simulink model "InnerOuter_Sim_newNav_flightgear_L2"  (Simulink 7.8)
settings: Solver=ode4  StartTime=0.0  StopTime=300  FixedStep=SampleT  RelTol=1e-3
InitFcn:
  | clc
  | innerOuterInit
  | launchFlightgear
values from neighbouring files (symbols this model uses):
  apSampleTime = 0.01    [innerOuterInit.m]
  FLIGHTGEAR_L2_RATE = 10    [launchFlightgear.m]
  SampleT = 0.005    [innerOuterInit.m]
  T = 0.01    [innerOuterInit.m]
undefined symbols (not defined in the file or in its folder): A1, Apolar, bankCommandLimit, baseHeight, BasePoint, baseTemp, CD0, chord, CL0, CLa, CLa_dot, Clb, ClDa, CLDe, CLDf, ClDr, clock, Clp, CLq, Clr, Cm0, Cma, CmDe, CmDf, Cmq, Cnb, CnDa, CnDr, Cnp, Cnr, compensatorOn, CYb, CYDr, da_failamp, da_failbias, da_failper, daL_fail, daR_fail, deg, DiscIntNeverNeededParam, dr_fail, dr_failamp, dr_failbias, dr_failper, Earth, elarm, Euler_0, F, gaind, getGSLocation, getWP, GS_location, Init_onlyOnce, Init_Reset, IPStar, ISA_g, Ixx, Iyy, Izz, L1OF ... (+38)
libraries: simulink x74, SLUGS_Library x41, aerolibconvert2 x24, dsPICdrivers x10, aerolibactuator x5, aerolibtransform2 x4, aerolibobsolete x3, dspmtrx3 x3, aerolibwind2 x2, aerolibfltsims x2, aerolibatmos2 x1, aerolibanimutils x1
(part 2 of 5)

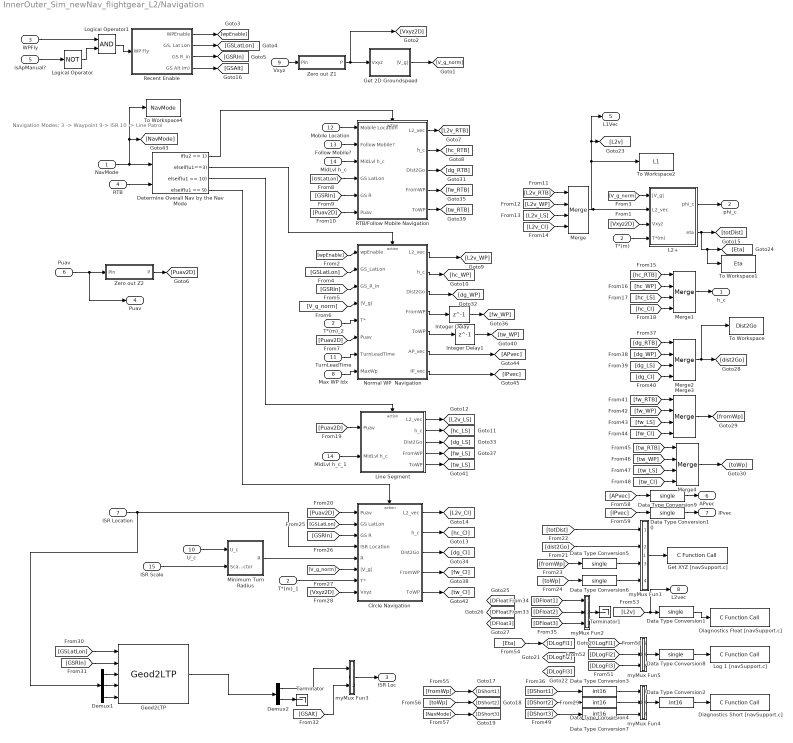
== system InnerOuter_Sim_newNav_flightgear_L2/Navigation ==
  note: Navigation Modes:
      | 3 -> Waypoint
      | 9-> ISR
      | 10 -> Line Patrol
  NavMode : Inport
  T*(m) : Inport  Port=2
  WPFly : Inport  Port=3
  RTB : Inport  Port=4
  isApManual? : Inport  Port=5
  Puav : Inport  Port=6  SampleTime=apSampleTime
  ISR Location : Inport  Port=7
  Max WP Idx : Inport  Port=8
  Vxyz : Inport  Port=9  SampleTime=apSampleTime
  U_c : Inport  Port=10
  TurnLeadTime : Inport  Port=11
  Mobile Location : Inport  Port=12
  Follow Mobile? : Inport  Port=13
  MidLvl h_c : Inport  Port=14
  ISR Scale : Inport  Port=15
  Circle Navigation : Subsystem  TreatAsAtomicUnit=on
  Data Type Conversion{1,5..6,8..10} (6 alike) : DataTypeConversion  OutDataTypeStr=single
  Data Type Conversion{2..4,7} (4 alike) : DataTypeConversion  OutDataTypeStr=int16
  Demux1 : Demux  Outputs=3
  Demux2 : Demux  Outputs=[2 1]
  Determine Overall Nav by the Nav Mode : If  NumInputs=2  IfExpression=u2 == 1  ElseIfExpressions=u1==3, u1 == 10, u1 == 9  ShowElse=off
  Diagnostics Float [navSupport.c] : dsPICdrivers/OTHERS/C Function Call  Tag=dsPIC_dsPIC_CFunctionCall  FctUpdate=Output Function  fctName='setDiagnosticFloat'  INPUT_SIZE=3  INPUT1=real32  INPUT2=--  INPUT3=--  OUTPUT_SIZE=1  OUTPUT1=--  SampleTime=.01  InputType=[ 7 ]  OutputType=[ ]  FctDeclaration=extern void setDiagnosticFloat(real32_T* u1);  FctCall=setDiagnosticFloat(*%u1);  OrderingInOutPopup=None  FctStart=None  FctStart_Name=Init_onlyOnce  FctStart_Declaration=inline extern void Init_onlyOnce();  FctStart_Call=Init_onlyOnce();  FctInit=None  FctInit_Name=Init_Reset  FctInit_Declaration=inline extern void Init_Reset();  FctInit_Call=Init_Reset();  PinDigitalInput=[]  PinDigitalOutput=[]  AnalogueInput=[]
  Diagnostics Short [navSupport.c] : dsPICdrivers/OTHERS/C Function Call  Tag=dsPIC_dsPIC_CFunctionCall  FctUpdate=Output Function  fctName='setDiagnosticShort'  INPUT_SIZE=3  INPUT1=int16  INPUT2=--  INPUT3=--  OUTPUT_SIZE=1  OUTPUT1=--  SampleTime=.01  InputType=[ 3 ]  OutputType=[ ]  FctDeclaration=extern void setDiagnosticShort(int16_T* u1);  FctCall=setDiagnosticShort(*%u1);  OrderingInOutPopup=None  FctStart=None  FctStart_Name=Init_onlyOnce  FctStart_Declaration=inline extern void Init_onlyOnce();  FctStart_Call=Init_onlyOnce();  FctInit=None  FctInit_Name=Init_Reset  FctInit_Declaration=inline extern void Init_Reset();  FctInit_Call=Init_Reset();  PinDigitalInput=[]  PinDigitalOutput=[]  AnalogueInput=[]
  Geod2LTP : SLUGS_Library/Navigation/Geod2LTP
  Get 2D Groundspeed : Subsystem
  Get XYZ [navSupport.c] : dsPICdrivers/OTHERS/C Function Call  Tag=dsPIC_dsPIC_CFunctionCall  FctUpdate=Output Function  fctName='setNavNav'  INPUT_SIZE=4  INPUT1=real32  INPUT2=--  INPUT3=--  OUTPUT_SIZE=1  OUTPUT1=--  SampleTime=.01  InputType=[ 7 ]  OutputType=[ ]  FctDeclaration=extern void setNavNav(real32_T* u1);  FctCall=setNavNav(*%u1);  OrderingInOutPopup=None  FctStart=None  FctStart_Name=Init_onlyOnce  FctStart_Declaration=inline extern void Init_onlyOnce();  FctStart_Call=Init_onlyOnce();  FctInit=None  FctInit_Name=Init_Reset  FctInit_Declaration=inline extern void Init_Reset();  FctInit_Call=Init_Reset();  PinDigitalInput=[]  PinDigitalOutput=[]  AnalogueInput=[]
  Integer Delay : Delay  DelayLength=1  InputProcessing=Inherited
  Integer Delay1 : Delay  DelayLength=1  InputProcessing=Inherited
  L2+ : Subsystem
  Line Segment : Subsystem  TreatAsAtomicUnit=on
  Log 1 [navSupport.c] : dsPICdrivers/OTHERS/C Function Call  Tag=dsPIC_dsPIC_CFunctionCall  FctUpdate=Output Function  fctName='setLogFloat1'  INPUT_SIZE=3  INPUT1=real32  INPUT2=--  INPUT3=--  OUTPUT_SIZE=1  OUTPUT1=--  SampleTime=.01  InputType=[ 7 ]  OutputType=[ ]  FctDeclaration=extern void setLogFloat1(real32_T* u1);  FctCall=setLogFloat1(*%u1);  OrderingInOutPopup=None  FctStart=None  FctStart_Name=Init_onlyOnce  FctStart_Declaration=inline extern void Init_onlyOnce();  FctStart_Call=Init_onlyOnce();  FctInit=None  FctInit_Name=Init_Reset  FctInit_Declaration=inline extern void Init_Reset();  FctInit_Call=Init_Reset();  PinDigitalInput=[]  PinDigitalOutput=[]  AnalogueInput=[]
  Logical Operator : Logic  Operator=NOT  AllPortsSameDT=off  OutDataTypeStr=boolean
  Logical Operator1 : Logic  AllPortsSameDT=off  OutDataTypeStr=boolean
  Merge{,1..4} (5 alike) : Merge  Inputs=4
  MidLvl h_c_1 : InportShadow  Port=14
  Minimum Turn Radius : Subsystem
  Normal WP  Navigation : Subsystem  TreatAsAtomicUnit=on
  RTB/Follow Mobile Navigation : Subsystem
  Recent Enable : Subsystem
  T*(m)_1 : InportShadow  Port=2
  T*(m)_2 : InportShadow  Port=2
  Terminator : Terminator
  Terminator1 : Terminator
  To Workspace : ToWorkspace  VariableName=Dist2Go  SampleTime=-1  SaveFormat=Array
  To Workspace1 : ToWorkspace  VariableName=Eta  SampleTime=-1  SaveFormat=Array
  To Workspace2 : ToWorkspace  VariableName=L1  SampleTime=-1  SaveFormat=Array
  To Workspace4 : ToWorkspace  VariableName=NavMode  SampleTime=-1  SaveFormat=Array
  Zero out Z1 : MATLAB Function  TreatAsAtomicUnit=on
  Zero out Z2 : MATLAB Function  TreatAsAtomicUnit=on
  myMux Fun1 : MATLAB Function  TreatAsAtomicUnit=on
  myMux Fun2 : MATLAB Function  TreatAsAtomicUnit=on
  myMux Fun3 : MATLAB Function  TreatAsAtomicUnit=on
  myMux Fun4 : MATLAB Function  TreatAsAtomicUnit=on
  myMux Fun5 : MATLAB Function  TreatAsAtomicUnit=on
  h_c : Outport
  phi_c : Outport  Port=2
  ISR Loc : Outport  Port=3
  "Puav " : Outport  Port=4
  L1Vec : Outport  Port=5
  APvec : Outport  Port=6
  IPvec : Outport  Port=7
  L2vec : Outport  Port=8
  wires:
  ? -> [DLogFl3]
  ? -> [DLogFl2]
  myMux Fun2/1(y) -> Terminator1/1
  ? -> [DFloat1]
  [NavMode] -> [DShort3]
  [toWp] -> [DShort2]
  [fromWp] -> [DShort1]
  [Eta] -> [DLogFl1]
  [L2v] -> Data Type Conversion1/1, L2vec/1
  Data Type Conversion8/1 -> Log 1 [navSupport.c]/1
  [DLogFl1] -> myMux Fun5/1(u1)
  [DLogFl2] -> myMux Fun5/2(u2)
  [DLogFl3] -> myMux Fun5/3(u3)
  myMux Fun5/1(y) -> Data Type Conversion8/1
  Data Type Conversion7/1 -> myMux Fun4/3(u3)
  Data Type Conversion4/1 -> myMux Fun4/2(u2)
  Data Type Conversion3/1 -> myMux Fun4/1(u1)
  [DShort3] -> Data Type Conversion7/1
  [DShort1] -> Data Type Conversion3/1
  [DShort2] -> Data Type Conversion4/1
  myMux Fun4/1(y) -> Data Type Conversion2/1
  Data Type Conversion2/1 -> Diagnostics Short [navSupport.c]/1
  [GSAlt] -> myMux Fun3/2(u2)
  Geod2LTP/1 -> Demux2/1
  Demux2/2 -> Terminator/1
  Demux2/1 -> myMux Fun3/1(u1)
  myMux Fun3/1(y) -> ISR Loc/1
  [GSRIn] -> Geod2LTP/2
  [GSLatLon] -> Geod2LTP/1
  Demux1/3 -> Geod2LTP/5
  Demux1/2 -> Geod2LTP/4
  Demux1/1 -> Geod2LTP/3
  Data Type Conversion1/1 -> Diagnostics Float [navSupport.c]/1
  [DFloat3] -> myMux Fun2/3(u3)
  [DFloat1] -> myMux Fun2/1(u1)
  [DFloat2] -> myMux Fun2/2(u2)
  ISR Scale/1 -> Minimum Turn Radius/2(Scale Factor)
  Recent Enable/4(GS Alt (m)) -> [GSAlt]
  Determine Overall Nav by the Nav Mode/3 -> Line Segment/Action
  U_c/1 -> Minimum Turn Radius/1(U_c)
  ISR Location/1 -> Demux1/1, Circle Navigation/4(ISR Location)
  [Vxyz2D] -> Circle Navigation/8(Vxyz)
  T*(m)_1/1 -> Circle Navigation/7(T*)
  [V_g_norm] -> Circle Navigation/6(|V_g|)
  Minimum Turn Radius/1(R) -> Circle Navigation/5(R)
  [GSRIn] -> Circle Navigation/3(GS R)
  [GSLatLon] -> Circle Navigation/2(GS LatLon)
  Circle Navigation/5(ToWP) -> [tw_CI]
  Circle Navigation/4(FromWP) -> [fw_CI]
  Circle Navigation/3(Dist2Go) -> [dg_CI]
  Circle Navigation/1(L2_vec) -> [L2v_CI]
  Circle Navigation/2(h_c) -> [hc_CI]
  [Puav2D] -> Circle Navigation/1(Puav)
  Integer Delay1/1 -> [tw_WP]
  Integer Delay/1 -> [fw_WP]
  Line Segment/5(ToWP) -> [tw_LS]
  RTB/Follow Mobile Navigation/5(ToWP) -> [tw_RTB]
  Line Segment/4(FromWP) -> [fw_LS]
  Normal WP  Navigation/4(FromWP) -> Integer Delay/1
  RTB/Follow Mobile Navigation/4(FromWP) -> [fw_RTB]
  Line Segment/3(Dist2Go) -> [dg_LS]
  Normal WP  Navigation/3(Dist2Go) -> [dg_WP]
  RTB/Follow Mobile Navigation/3(Dist2Go) -> [dg_RTB]
  Merge3/1 -> [fromWp]
  Merge4/1 -> [toWp]
  Merge2/1 -> [dist2Go], To Workspace/1
  [tw_RTB] -> Merge4/1
  [tw_WP] -> Merge4/2
  [tw_LS] -> Merge4/3
  [tw_CI] -> Merge4/4
  [fw_RTB] -> Merge3/1
  [fw_WP] -> Merge3/2
  [fw_LS] -> Merge3/3
  [fw_CI] -> Merge3/4
  [dg_RTB] -> Merge2/1
  [dg_WP] -> Merge2/2
  [dg_LS] -> Merge2/3
  [dg_CI] -> Merge2/4
  L2+/2(eta) -> [totDist], [Eta], To Workspace1/1
  Data Type Conversion6/1 -> myMux Fun1/4(u4)
  Data Type Conversion5/1 -> myMux Fun1/3(u3)
  [toWp] -> Data Type Conversion6/1
  [fromWp] -> Data Type Conversion5/1
  [dist2Go] -> myMux Fun1/2(u2)
  [totDist] -> myMux Fun1/1(u1)
  myMux Fun1/1(y) -> Get XYZ [navSupport.c]/1
  Vxyz/1 -> Zero out Z1/1(Pin)
  Get 2D Groundspeed/1(|V_g|) -> [V_g_norm]
  [Vxyz2D] -> L2+/3(Vxyz)
  [V_g_norm] -> L2+/1(|V_g|)
  L2+/1(phi_c) -> phi_c/1
  T*(m)/1 -> L2+/4(T*(m))
  NavMode/1 -> Determine Overall Nav by the Nav Mode/1, [NavMode], To Workspace4/1
  Merge/1 -> L2+/2(L2_vec), To Workspace2/1, [L2v], L1Vec/1
  Recent Enable/1(WPEnable) -> [wpEnable]
  Recent Enable/2("GS, Lat Lon") -> [GSLatLon]
  Recent Enable/3(GS R_in) -> [GSRIn]
  Determine Overall Nav by the Nav Mode/2 -> Normal WP  Navigation/Action
  Determine Overall Nav by the Nav Mode/4 -> Circle Navigation/Action
  RTB/1 -> Determine Overall Nav by the Nav Mode/2
  Follow Mobile?/1 -> RTB/Follow Mobile Navigation/2(Follow Mobile?)
  MidLvl h_c/1 -> RTB/Follow Mobile Navigation/3(MidLvl h_c)
  Mobile Location/1 -> RTB/Follow Mobile Navigation/1(Mobile Location)
  Determine Overall Nav by the Nav Mode/1 -> RTB/Follow Mobile Navigation/Action
  Zero out Z1/1(P) -> Get 2D Groundspeed/1(Vxyz), [Vxyz2D]
  Puav/1 -> "Puav "/1, Zero out Z2/1(Pin)
  [GSRIn] -> Normal WP  Navigation/3(GS_R_in)
  [GSLatLon] -> Normal WP  Navigation/2(GS_LatLon)
  [wpEnable] -> Normal WP  Navigation/1(wpEnable)
  [V_g_norm] -> Normal WP  Navigation/4(|V_g|)
  T*(m)_2/1 -> Normal WP  Navigation/5(T*)
  [Puav2D] -> Normal WP  Navigation/6(Puav)
  TurnLeadTime/1 -> Normal WP  Navigation/7(TurnLeadTime)
  Max WP Idx/1 -> Normal WP  Navigation/8(MaxWp)
  [GSLatLon] -> RTB/Follow Mobile Navigation/4(GS LatLon)
  [GSRIn] -> RTB/Follow Mobile Navigation/5(GS R)
  Zero out Z2/1(P) -> [Puav2D]
  [Puav2D] -> RTB/Follow Mobile Navigation/6(Puav)
  Merge1/1 -> h_c/1
  RTB/Follow Mobile Navigation/1(L2_vec) -> [L2v_RTB]
  RTB/Follow Mobile Navigation/2(h_c) -> [hc_RTB]
  Normal WP  Navigation/1(L2_vec) -> [L2v_WP]
  Normal WP  Navigation/2(h_c) -> [hc_WP]
  Line Segment/1(L2_vec) -> [L2v_LS]
  Line Segment/2(h_c) -> [hc_LS]
  [L2v_RTB] -> Merge/1
  [L2v_WP] -> Merge/2
  [L2v_LS] -> Merge/3
  [L2v_CI] -> Merge/4
  [hc_RTB] -> Merge1/1
  [hc_WP] -> Merge1/2
  [hc_LS] -> Merge1/3
  [hc_CI] -> Merge1/4
  [Puav2D] -> Line Segment/1(Puav)
  MidLvl h_c_1/1 -> Line Segment/2(MidLvl h_c)
  isApManual?/1 -> Logical Operator/1
  Logical Operator1/1 -> Recent Enable/1(WP Fly)
  Logical Operator/1 -> Logical Operator1/2
  WPFly/1 -> Logical Operator1/1
  Normal WP  Navigation/5(ToWP) -> Integer Delay1/1
  Normal WP  Navigation/6(AP_vec) -> [APvec]
  [APvec] -> Data Type Conversion9/1
  Data Type Conversion9/1 -> APvec/1
  Normal WP  Navigation/7(IP_vec) -> [IPvec]
  [IPvec] -> Data Type Conversion10/1
  Data Type Conversion10/1 -> IPvec/1

== system InnerOuter_Sim_newNav_flightgear_L2/PT Unit (Mariano) ==
  Rb2g : Inport
  cor_b : Inport  Port=2
  Puav : Inport  Port=3
  ISR Location : Inport  Port=4
  Divide : Product  Inputs=*/
  Normalize : Product  Inputs=*/
  Product1 : Product  Multiplication=Matrix(*)  RndMeth=Zero
  Product2 : Product  Multiplication=Matrix(*)  RndMeth=Zero
  Subtract2 : Sum  Inputs=--+
  Transpose1 : dspmtrx3/Transpose  Hermitian=off  overflowFlag=off
  Vector Norm : SLUGS_Library/Vector Norm
  "[-90 90]" : Saturate  UpperLimit=1.5708  LowerLimit=-1.5708
  "[-90 90]1" : Saturate  UpperLimit=1.5708  LowerLimit=-1.5708
  "[a b c]" : Demux  Outputs=3
  dsPIC_asin : SLUGS_Library/dsPIC_asin
  dsPIC_atan : SLUGS_Library/dsPIC_atan
  Tilt_c : Outport
  Pan_c : Outport  Port=2
  wires:
  Rb2g/1 -> Transpose1/1, Product2/1  "Tbg"
  cor_b/1 -> Product1/2
  Vector Norm/1 -> Normalize/2
  Normalize/1 -> Product2/2
  Product2/1 -> "[a b c]"/1
  "[a b c]"/3 -> dsPIC_asin/1
  "[a b c]"/2 -> Divide/1
  "[a b c]"/1 -> Divide/2
  Divide/1 -> dsPIC_atan/1
  dsPIC_atan/1 -> "[-90 90]"/1
  Subtract2/1 -> Normalize/1, Vector Norm/1
  Transpose1/1 -> Product1/1
  "[-90 90]"/1 -> Pan_c/1
  "[-90 90]1"/1 -> Tilt_c/1
  dsPIC_asin/1 -> "[-90 90]1"/1
  ISR Location/1 -> Subtract2/3  "Xt"
  Puav/1 -> Subtract2/2  "Xac"
  Product1/1 -> Subtract2/1  "Tgb * cor_b"

== system InnerOuter_Sim_newNav_flightgear_L2/PT Unit (Vlad)  ==
  Euler (Rad) : Inport
  Tgt (NEU) : Inport  Port=2
  Puav (NEU) : Inport  Port=3
  Display1 : Display
  Divide : Product  Inputs=*/
  LPF the Euler and Construct Matrix : Subsystem
  Product1 : Product  Multiplication=Matrix(*)  RndMeth=Zero
  Subtract : Sum  Inputs=+-
  Trigonometric Function1 : Trigonometry  Operator=atan2
  Trigonometric Function2 : Trigonometry  Operator=asin
  Vector Norm : SLUGS_Library/Vector Norm
  "[-1 1]" : Saturate  UpperLimit=1  LowerLimit=-1
  "[-88 0]" : Saturate  UpperLimit=0  LowerLimit=-1.5708
  "[-98 98]" : Saturate  UpperLimit=1.7104  LowerLimit=-1.7104
  "[a b c]" : Demux  Outputs=3
  Tilt (rad) : Outport
  Pan (rad) : Outport  Port=2
  wires:
  Subtract/1 -> Product1/2  "Tgt_WR_UAV  (NEU)"
  LPF the Euler and Construct Matrix/1(Rfg2b) -> Product1/1
  "[a b c]"/2 -> Trigonometric Function1/1
  "[a b c]"/1 -> Trigonometric Function1/2
  Trigonometric Function1/1 -> "[-98 98]"/1
  Trigonometric Function2/1 -> "[-88 0]"/1, Display1/1
  Product1/1 -> "[a b c]"/1, Vector Norm/1
  "[-1 1]"/1 -> Trigonometric Function2/1
  "[a b c]"/3 -> Divide/1
  Vector Norm/1 -> Divide/2
  Divide/1 -> "[-1 1]"/1
  Euler (Rad)/1 -> LPF the Euler and Construct Matrix/1(Euler)
  "[-98 98]"/1 -> Pan (rad)/1
  Tgt (NEU)/1 -> Subtract/1
  "[-88 0]"/1 -> Tilt (rad)/1
  Puav (NEU)/1 -> Subtract/2

== system InnerOuter_Sim_newNav_flightgear_L2/Send IP to Flightgear ==
  IPvec : Inport
  Enable : EnablePort
  Demux8 : Demux  Outputs=2
  First WP Height : Constant  Value=Zpoints(1)  SampleTime=-1
  Flat Earth to LLA1 : aerolibtransform2/Flat Earth to LLA  units=Metric (MKS)  ptype=Earth (WGS84)  F=1/298.257223563  R=6378137  LL0=GS_location(2:3)  psi=0
  MATLAB Function : MATLAB Function  TreatAsAtomicUnit=on
  NEU2NED : Gain  Gain=[ 1 1 -1]'  SaturateOnIntegerOverflow=on  OutDataTypeStr=Inherit: Same as input  ParamDataTypeStr=Inherit: Same as input
  Terminator : Terminator
  Zero level trust : Constant  Value=0  SampleTime=-1
  wires:
  NEU2NED/1 -> Flat Earth to LLA1/1
  Zero level trust/1 -> Flat Earth to LLA1/2
  Demux8/1 -> MATLAB Function/1(ip_lat)
  Demux8/2 -> MATLAB Function/2(ip_lon)
  Flat Earth to LLA1/1 -> Demux8/1
  Flat Earth to LLA1/2 -> Terminator/1
  First WP Height/1 -> MATLAB Function/3(ip_h)
  IPvec/1 -> NEU2NED/1

== system InnerOuter_Sim_newNav_flightgear_L2/Send L2 to Flightgear ==
  L2vec : Inport
  Enable : EnablePort
  Demux : Demux  Outputs=3
  Demux8 : Demux  Outputs=2
  Flat Earth to LLA1 : aerolibtransform2/Flat Earth to LLA  units=Metric (MKS)  ptype=Earth (WGS84)  F=1/298.257223563  R=6378137  LL0=GS_location(2:3)  psi=0
  MATLAB Function : MATLAB Function  TreatAsAtomicUnit=on
  Mux : Mux  Inputs=3
  NEU2NED : Gain  Gain=[ 1 1 -1]'  SaturateOnIntegerOverflow=on  OutDataTypeStr=Inherit: Same as input  ParamDataTypeStr=Inherit: Same as input
  Terminator : Terminator
  Zero level trust : Constant  Value=0  SampleTime=-1
  wires:
  NEU2NED/1 -> Flat Earth to LLA1/1
  Zero level trust/1 -> Flat Earth to LLA1/2
  Flat Earth to LLA1/1 -> Demux8/1
  Flat Earth to LLA1/2 -> Terminator/1
  Demux8/2 -> MATLAB Function/2(l2_lon)
  Demux8/1 -> MATLAB Function/1(l2_lat)
  Demux/3 -> Mux/3
  L2vec/1 -> Demux/1
  Mux/1 -> NEU2NED/1
  Demux/1 -> Mux/1
  Demux/2 -> Mux/2

== system InnerOuter_Sim_newNav_flightgear_L2/Simple Car Model ==
  Heading : Inport
  Speed : Inport  Port=2
  Heading/Speed to Velocity : Subsystem
  Simple Car Model : Subsystem
  basePoint : Outport
  wires:
  Heading/Speed to Velocity/1(Velocity) -> Simple Car Model/1(Velocity)
  Heading/1 -> Heading/Speed to Velocity/1(Heading)
  Simple Car Model/1(p_cg) -> basePoint/1
  Speed/1 -> Heading/Speed to Velocity/2(Speed)

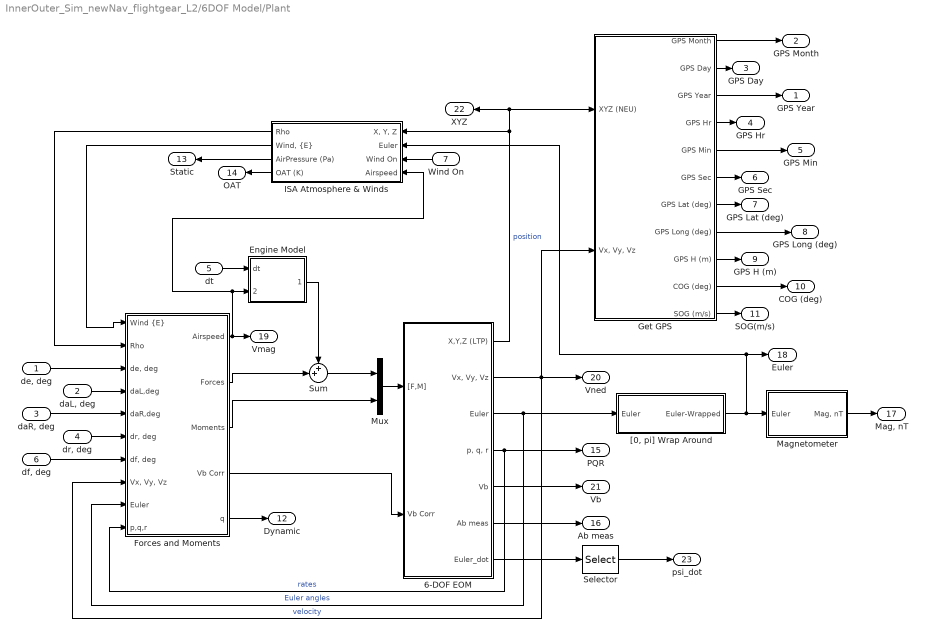
== system InnerOuter_Sim_newNav_flightgear_L2/6DOF Model/Plant ==
  "de, deg" : Inport
  "daL, deg" : Inport  Port=2
  "daR, deg" : Inport  Port=3
  "dr, deg" : Inport  Port=4
  dt : Inport  Port=5
  "df, deg" : Inport  Port=6
  Wind On : Inport  Port=7
  6-DOF EOM : Subsystem
  Engine Model : Subsystem
  Forces and Moments : Subsystem
  Get GPS : Subsystem
  ISA Atmosphere & Winds : Subsystem
  Magnetometer : Subsystem  mask{magField=[ 23143.6 5858.2 45511.9]}
      mask prompts: magField "Local Magnetic Field"
      mask help:
      | Simulates the Data from magnetometers with no noise.
      |
      | You can obtain data for the local magnetic field at:
      |
      | http://www.ngdc.noaa.gov/geomagmodels/IGRFWMM.jsp
  Mux : Mux  Inputs=2
  Selector : Selector  InputPortWidth=3  IndexOptions=Index vector (dialog)  Indices=[3]  OutputSizes=1
  Sum : Sum  Inputs=++|  SaturateOnIntegerOverflow=on
  "[0, pi] Wrap Around" : Subsystem
  GPS Year : Outport
  GPS Month : Outport  Port=2
  GPS Day : Outport  Port=3
  GPS Hr : Outport  Port=4
  GPS Min : Outport  Port=5
  GPS Sec : Outport  Port=6
  GPS Lat (deg) : Outport  Port=7
  GPS Long (deg) : Outport  Port=8
  GPS H (m) : Outport  Port=9
  COG (deg) : Outport  Port=10
  SOG(m/s) : Outport  Port=11
  Dynamic : Outport  Port=12
  Static : Outport  Port=13
  OAT : Outport  Port=14
  PQR : Outport  Port=15
  Ab meas : Outport  Port=16
  "Mag, nT" : Outport  Port=17
  Euler : Outport  Port=18
  Vmag : Outport  Port=19
  Vned : Outport  Port=20
  Vb : Outport  Port=21
  XYZ : Outport  Port=22
  psi_dot : Outport  Port=23
  wires:
  Get GPS/1(GPS Month) -> GPS Month/1
  Get GPS/2(GPS Day) -> GPS Day/1
  Get GPS/3(GPS Year) -> GPS Year/1
  Get GPS/4(GPS Hr) -> GPS Hr/1
  Get GPS/5(GPS Min) -> GPS Min/1
  Get GPS/6(GPS Sec) -> GPS Sec/1
  Get GPS/7(GPS Lat (deg)) -> GPS Lat (deg)/1
  Get GPS/8(GPS Long (deg)) -> GPS Long (deg)/1
  Get GPS/9(GPS H (m)) -> GPS H (m)/1
  6-DOF EOM/6(Ab meas) -> Ab meas/1
  Mux/1 -> 6-DOF EOM/1("[F,M]")
  6-DOF EOM/5(Vb) -> Vb/1
  Engine Model/1(Thrust) -> Sum/1
  Forces and Moments/5(q) -> Dynamic/1
  ISA Atmosphere & Winds/3(AirPressure (Pa)) -> Static/1
  Forces and Moments/1(Airspeed) -> Vmag/1, Engine Model/2(Vmag), ISA Atmosphere & Winds/4(Airspeed)
  ISA Atmosphere & Winds/2("Wind, {E}") -> Forces and Moments/1("Wind {E}")
  ISA Atmosphere & Winds/1(Rho) -> Forces and Moments/2(Rho)
  Forces and Moments/3(Moments) -> Mux/2
  Forces and Moments/2(Forces) -> Sum/2
  Sum/1 -> Mux/1
  Forces and Moments/4(Vb Corr) -> 6-DOF EOM/2(Vb Corr)
  6-DOF EOM/1(X,Y,Z (LTP)) -> ISA Atmosphere & Winds/1("X, Y, Z"), Get GPS/1(XYZ (NEU)), XYZ/1  "position"
  6-DOF EOM/2("Vx, Vy, Vz") -> Vned/1, Get GPS/2("Vx, Vy, Vz"), Forces and Moments/8("Vx, Vy, Vz ")  "velocity"
  6-DOF EOM/3(Euler) -> "[0, pi] Wrap Around"/1(Euler), Forces and Moments/9(Euler)  "Euler angles"
  6-DOF EOM/4("p, q, r") -> PQR/1, Forces and Moments/10(p,q,r)  "rates"
  dt/1 -> Engine Model/1(dt)
  "de, deg"/1 -> Forces and Moments/3("de, deg")
  "daL, deg"/1 -> Forces and Moments/4(daL,deg)
  "dr, deg"/1 -> Forces and Moments/6("dr, deg")
  "df, deg"/1 -> Forces and Moments/7("df, deg")
  "[0, pi] Wrap Around"/1(Euler-Wrapped) -> Magnetometer/1(Euler), Euler/1, ISA Atmosphere & Winds/2(Euler)
  Magnetometer/1("Mag, nT") -> "Mag, nT"/1
  Get GPS/10(COG (deg)) -> COG (deg)/1
  Get GPS/11(SOG (m/s)) -> SOG(m/s)/1
  ISA Atmosphere & Winds/4(OAT (K)) -> OAT/1
  6-DOF EOM/7(Euler_dot) -> Selector/1
  Selector/1 -> psi_dot/1
  Wind On/1 -> ISA Atmosphere & Winds/3(Wind On)
  "daR, deg"/1 -> Forces and Moments/5(daR,deg)

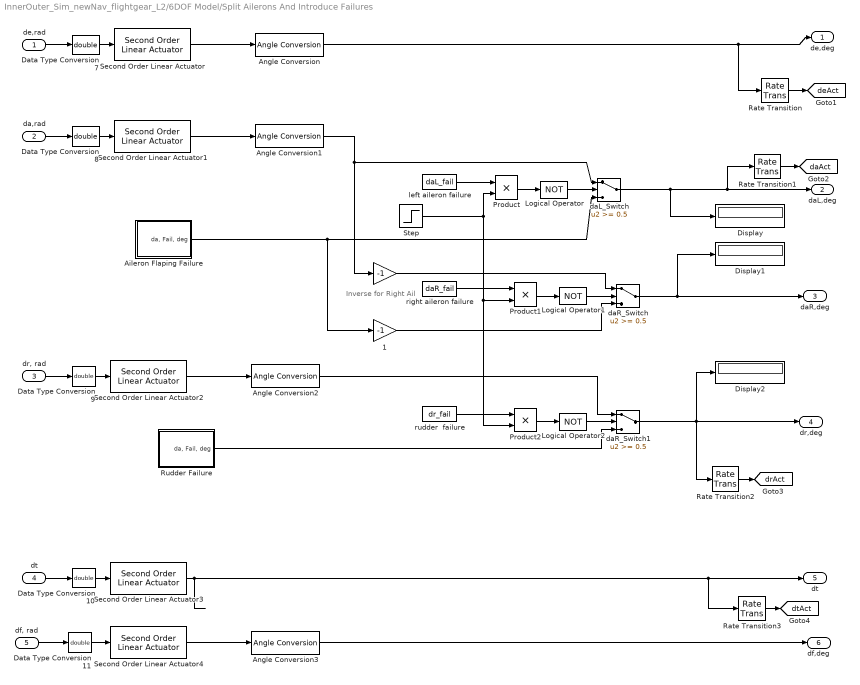
== system InnerOuter_Sim_newNav_flightgear_L2/6DOF Model/Split Ailerons And Introduce Failures ==
  note: Inverse
      | for Right
      | Ail
  de,rad : Inport
  da,rad : Inport  Port=2
  "dr, rad" : Inport  Port=3
  dt : Inport  Port=4
  "df, rad" : Inport  Port=5
  " " : Gain  Gain=-1  SaturateOnIntegerOverflow=on  OutDataTypeStr=Inherit: Same as input  ParamDataTypeStr=Inherit: Same as input
  " 1" : Gain  Gain=-1  SaturateOnIntegerOverflow=on  OutDataTypeStr=Inherit: Same as input  ParamDataTypeStr=Inherit: Same as input
  Aileron Flaping Failure : Subsystem
  Angle Conversion{,1..3} (4 alike) : aerolibconvert2/Angle Conversion  IU=rad  OU=deg
  Data Type Conversion{7..11} (5 alike) : DataTypeConversion  OutDataTypeStr=double
  Display : Display
  Display1 : Display
  Display2 : Display
  Logical Operator : Logic  Operator=NOT  AllPortsSameDT=off  OutDataTypeStr=boolean
  Logical Operator1 : Logic  Operator=NOT  AllPortsSameDT=off  OutDataTypeStr=boolean
  Logical Operator2 : Logic  Operator=NOT  AllPortsSameDT=off  OutDataTypeStr=boolean
  Product : Product  RndMeth=Zero
  Product1 : Product  RndMeth=Zero
  Product2 : Product  RndMeth=Zero
  Rate Transition{,1..3} (4 alike) : RateTransition  OutPortSampleTime=apSampleTime
  Rudder Failure : Subsystem
  Second Order Linear Actuator{,1..3} (4 alike) : aerolibactuator/Second Order Linear Actuator  wn_fin=15  z_fin=0.8  fin_act_0=0
  Second Order Linear Actuator4 : aerolibactuator/Second Order Linear Actuator  wn_fin=150  z_fin=0.7  fin_act_0=0
  Step : Step  Time=tfailure
  daL_Switch : Switch  Threshold=0.5
  daR_Switch : Switch  Threshold=0.5
  daR_Switch1 : Switch  Threshold=0.5
  left aileron failure : Constant  Value=daL_fail
  right aileron failure : Constant  Value=daR_fail
  rudder  failure : Constant  Value=dr_fail
  de,deg : Outport
  daL,deg : Outport  Port=2
  daR,deg : Outport  Port=3
  dr,deg : Outport  Port=4
  "dt " : Outport  Port=5
  df,deg : Outport  Port=6
  tag scope: daAct=global, deAct=global, drAct=global, dtAct=global
  wires:
  de,rad/1 -> Data Type Conversion7/1
  da,rad/1 -> Data Type Conversion8/1
  "dr, rad"/1 -> Data Type Conversion9/1
  dt/1 -> Data Type Conversion10/1
  "df, rad"/1 -> Data Type Conversion11/1
  Second Order Linear Actuator/1 -> Angle Conversion/1
  Second Order Linear Actuator1/1 -> Angle Conversion1/1
  Second Order Linear Actuator2/1 -> Angle Conversion2/1
  Second Order Linear Actuator3/1 -> "dt "/1, Rate Transition3/1
  Second Order Linear Actuator4/1 -> Angle Conversion3/1
  Rate Transition1/1 -> [daAct]
  Rate Transition2/1 -> [drAct]
  Rate Transition3/1 -> [dtAct]
  Data Type Conversion7/1 -> Second Order Linear Actuator/1
  Data Type Conversion8/1 -> Second Order Linear Actuator1/1
  Data Type Conversion9/1 -> Second Order Linear Actuator2/1
  Data Type Conversion10/1 -> Second Order Linear Actuator3/1
  Data Type Conversion11/1 -> Second Order Linear Actuator4/1
  Angle Conversion/1 -> de,deg/1, Rate Transition/1
  Angle Conversion1/1 -> daL_Switch/1, " "/1
  Angle Conversion2/1 -> daR_Switch1/1
  Angle Conversion3/1 -> df,deg/1
  left aileron failure/1 -> Product/1
  Aileron Flaping Failure/1("da, Fail, deg") -> daL_Switch/3, " 1"/1
  Product/1 -> Logical Operator/1
  Logical Operator/1 -> daL_Switch/2
  Step/1 -> Product/2, Product1/2, Product2/2
  daL_Switch/1 -> Display/1, daL,deg/1, Rate Transition1/1
  right aileron failure/1 -> Product1/1
  Product1/1 -> Logical Operator1/1
  Logical Operator1/1 -> daR_Switch/2
  " "/1 -> daR_Switch/1
  " 1"/1 -> daR_Switch/3
  daR_Switch/1 -> daR,deg/1, Display1/1
  rudder  failure/1 -> Product2/1
  Product2/1 -> Logical Operator2/1
  Logical Operator2/1 -> daR_Switch1/2
  daR_Switch1/1 -> dr,deg/1, Display2/1, Rate Transition2/1
  Rate Transition/1 -> [deAct]
  Rudder Failure/1("da, Fail, deg") -> daR_Switch1/3

== system InnerOuter_Sim_newNav_flightgear_L2/6DOF Model/Subsystem ==
  Signal In : Inport
  Noise On : Inport  Port=2
  Add : Sum
  Random Number : RandomNumber  Variance=nv  Seed=ns  SampleTime=st
  Signal1 : InportShadow  Port=1
  Switch : Switch  Threshold=0.3
  Signal Out : Outport
  wires:
  Random Number/1 -> Add/2
  Add/1 -> Switch/1
  Signal In/1 -> Add/1
  Noise On/1 -> Switch/2
  Switch/1 -> Signal Out/1
  Signal1/1 -> Switch/3

== system InnerOuter_Sim_newNav_flightgear_L2/6DOF Model/Subsystem1 ==
  Signal In : Inport
  Noise On : Inport  Port=2
  Add : Sum
  Random Number : RandomNumber  Variance=nv  Seed=ns  SampleTime=st
  Signal1 : InportShadow  Port=1
  Switch : Switch  Threshold=0.3
  Signal Out : Outport
  wires:
  Signal1/1 -> Switch/3
  Switch/1 -> Signal Out/1
  Noise On/1 -> Switch/2
  Signal In/1 -> Add/1
  Add/1 -> Switch/1
  Random Number/1 -> Add/2

== system InnerOuter_Sim_newNav_flightgear_L2/6DOF Model/Subsystem2 ==
  Signal In : Inport
  Noise On : Inport  Port=2
  Add : Sum
  Random Number : RandomNumber  Variance=nv  Seed=ns  SampleTime=st
  Signal1 : InportShadow  Port=1
  Switch : Switch  Threshold=0.3
  Signal Out : Outport
  wires:
  Random Number/1 -> Add/2
  Add/1 -> Switch/1
  Signal In/1 -> Add/1
  Noise On/1 -> Switch/2
  Switch/1 -> Signal Out/1
  Signal1/1 -> Switch/3

== system InnerOuter_Sim_newNav_flightgear_L2/6DOF Model/Subsystem3 ==
  Signal In : Inport
  Noise On : Inport  Port=2
  Add : Sum
  Random Number : RandomNumber  Variance=nv  Seed=ns  SampleTime=st
  Signal1 : InportShadow  Port=1
  Switch : Switch  Threshold=0.3
  Signal Out : Outport
  wires:
  Signal1/1 -> Switch/3
  Switch/1 -> Signal Out/1
  Noise On/1 -> Switch/2
  Signal In/1 -> Add/1
  Add/1 -> Switch/1
  Random Number/1 -> Add/2

== system InnerOuter_Sim_newNav_flightgear_L2/6DOF Model/Subsystem4 ==
  Signal In : Inport
  Noise On : Inport  Port=2
  Add : Sum
  Random Number : RandomNumber  Variance=nv  Seed=ns  SampleTime=st
  Signal1 : InportShadow  Port=1
  Switch : Switch  Threshold=0.3
  Signal Out : Outport
  wires:
  Signal1/1 -> Switch/3
  Switch/1 -> Signal Out/1
  Noise On/1 -> Switch/2
  Signal In/1 -> Add/1
  Add/1 -> Switch/1
  Random Number/1 -> Add/2

== system InnerOuter_Sim_newNav_flightgear_L2/6DOF Model/Subsystem5 ==
  Signal In : Inport
  Noise On : Inport  Port=2
  Add : Sum
  Random Number : RandomNumber  Variance=nv  Seed=ns  SampleTime=st
  Signal1 : InportShadow  Port=1
  Switch : Switch  Threshold=0.3
  Signal Out : Outport
  wires:
  Random Number/1 -> Add/2
  Add/1 -> Switch/1
  Signal In/1 -> Add/1
  Noise On/1 -> Switch/2
  Switch/1 -> Signal Out/1
  Signal1/1 -> Switch/3

== system InnerOuter_Sim_newNav_flightgear_L2/6DOF Model/Subsystem6 ==
  Signal In : Inport
  Noise On : Inport  Port=2
  Add : Sum
  Random Number : RandomNumber  Variance=nv  Seed=ns  SampleTime=st
  Signal1 : InportShadow  Port=1
  Switch : Switch  Threshold=0.3
  Signal Out : Outport
  wires:
  Signal1/1 -> Switch/3
  Switch/1 -> Signal Out/1
  Noise On/1 -> Switch/2
  Signal In/1 -> Add/1
  Add/1 -> Switch/1
  Random Number/1 -> Add/2

== system InnerOuter_Sim_newNav_flightgear_L2/Bank to Psi Dot/Subsystem8 ==
  x : Inport
  C Function Call1 : dsPICdrivers/OTHERS/C Function Call  Tag=dsPIC_dsPIC_CFunctionCall  FctUpdate=Output Function  fctName='myTan'  INPUT_SIZE=1  INPUT1=real32  INPUT2=--  INPUT3=--  OUTPUT_SIZE=1  OUTPUT1=real32  SampleTime=-1  InputType=[ 7 ]  OutputType=[ 7 ]  FctDeclaration=extern real32_T myTan(real32_T u1);  FctCall=%y1 = myTan(%u1);  OrderingInOutPopup=None  FctStart=None  FctStart_Name=Init_onlyOnce  FctStart_Declaration=inline extern void Init_onlyOnce();  FctStart_Call=Init_onlyOnce();  FctInit=None  FctInit_Name=Init_Reset  FctInit_Declaration=inline extern void Init_Reset();  FctInit_Call=Init_Reset();  PinDigitalInput=[]  PinDigitalOutput=[]  AnalogueInput=[]
  Environment Controller : simulink/Signal Routing/Environment Controller
  Trigonometric Function : Trigonometry  Operator=tan
  tan(x) : Outport
  wires:
  Environment Controller/1 -> tan(x)/1
  C Function Call1/1 -> Environment Controller/2
  Trigonometric Function/1 -> Environment Controller/1
  x/1 -> Trigonometric Function/1, C Function Call1/1

== system InnerOuter_Sim_newNav_flightgear_L2/BaroTest/Compute Barometric Height ==
  Base Height (m) : Inport
  Base Pressure (Pa) : Inport  Port=2
  Baro (Pa) : Inport  Port=3
  Constant2 : Constant  Value=baseTemp/(-LapseRate)  OutDataTypeStr=single
  Constant3 : Constant  Value=9.350253e-2  OutDataTypeStr=single
  Constant4 : Constant  Value=-1.888933e-1  OutDataTypeStr=single
  Constant5 : Constant  Value=2.180313e-5  OutDataTypeStr=single
  Divide : Product  Inputs=*/  OutDataTypeStr=single
  Divide{1..4} (4 alike) : Product  OutDataTypeStr=single
  Length Conversion : aerolibconvert2/Length Conversion  IU=ft  OU=m
  Sum1 : Sum  Inputs=|++  OutDataTypeStr=single
  Sum2 : Sum  Inputs=|+-  OutDataTypeStr=single
  Sum3 : Sum  Inputs=3  OutDataTypeStr=single
  "Altitude, m" : Outport
  wires:
  Length Conversion/1 -> Sum1/1
  Sum2/1 -> Divide/1
  Sum1/1 -> "Altitude, m"/1
  Divide3/1 -> Length Conversion/1
  Constant2/1 -> Divide3/2
  Sum3/1 -> Divide3/1
  Constant5/1 -> Sum3/3
  Divide2/1 -> Sum3/2
  Divide1/1 -> Sum3/1
  Constant4/1 -> Divide2/2
  Constant3/1 -> Divide1/2
  Divide4/1 -> Divide1/1  "x^2"
  Divide/1 -> Divide2/1, Divide4/1, Divide4/2  "x"
  Base Pressure (Pa)/1 -> Divide/2, Sum2/2
  Base Height (m)/1 -> Sum1/2
  Baro (Pa)/1 -> Sum2/1

== system InnerOuter_Sim_newNav_flightgear_L2/BaroTest/Initial Baro Bias ==
  Baro (Pa) : Inport
  Enable : EnablePort
  Data Type Conversion : DataTypeConversion  OutDataTypeStr=double
  Data Type Conversion1 : DataTypeConversion  OutDataTypeStr=single
  Low Pass8 : Subsystem  mask(DiscretizedZeroPole){Zeros=[], Poles=[-3], Gain=3, AbsTol=auto, SampleTime=.01, method=tustin, Wc=1}
      mask prompts: Zeros "Zeros (enter in s-main:)"; Poles "Poles (enter in s-domain:)"; Gain "Gain (enter in s-domain:)"; AbsTol "Absolute tolerance:"; SampleTime "Sample time:"; Wc "Critical Frequency (Hz):"
      mask help: Continuous mask uses c2d to transform parameters onto the Discrete Zero-Pole block inside.
      mask init:
      | st=SampleTime;
      | if length(st)>1
      |     st=SampleTime(1);
      | end
      | if(st>0)
      |     [zerosd,polesd,gaind] = sldiscutil('disczpk', {st,method,Wc,Zeros,Poles,Gain});
      | end	
      | s = get_param(gcb,'maskvalues');
      | zeross = s{1};
      | poless = s{2};
      | gainss = s{3};
      | %zerosc = eval(zeross);
      | %polesc = eval(poless);
      | %gainsc = eval(gainss);
      | sldiscutil('initzpkmask', st);
      | if(st==0)
      | set_param([gcb '/Zero Pole'], 'AbsoluteTolerance', AbsTol);
      | end
      mask StyleString: edit,edit,edit,edit,edit,popup(zoh|foh|tustin|prewarp|matched),edit
      mask CallbackString: |||||hidecrit|
      mask Display:
      | droots(zeross,poless,gainss)
      | text( 0.5, 1.0, method, 'verticalAlignment','top')
  Mux : Mux  Inputs=2
  Scope : Scope
      settings: SaveName=ScopeData8
  "[80k - 120k]" : Saturate  UpperLimit=120000  LowerLimit=80000
  Baro (Gnd) : Outport
  wires:
  Baro (Pa)/1 -> Data Type Conversion/1
  Low Pass8/1(Out1) -> Data Type Conversion1/1
  Data Type Conversion/1 -> Low Pass8/1(In1)
  Data Type Conversion1/1 -> Mux/2, "[80k - 120k]"/1
  Mux/1 -> Scope/1
  "[80k - 120k]"/1 -> Baro (Gnd)/1, Mux/1

== system InnerOuter_Sim_newNav_flightgear_L2/BaroTest/Zero Out Height ==
  Base Height : Inport
  Computed Height : Inport  Port=2
  Enable : EnablePort
  Integer Delay : Delay  DelayLength=1  InitialCondition=0  InputProcessing=Inherited  SampleTime=.01
  Sum : Sum  Inputs=|+-  OutDataTypeStr=single
  Height Offset : Outport
  wires:
  Computed Height/1 -> Integer Delay/1
  Sum/1 -> Height Offset/1
  Integer Delay/1 -> Sum/2
  Base Height/1 -> Sum/1

== system InnerOuter_Sim_newNav_flightgear_L2/Create ISR Location From WPs/get sim WP Coord from Index ==
  WP Idx : Inport
  Data Type Conversion : DataTypeConversion  OutDataTypeStr=double
  Data Type Conversion1 : DataTypeConversion  OutDataTypeStr=single
  MATLAB Fcn : MATLABFcn  MATLABFcn=Xpoints(u(1))  OutputDimensions=1  OutputSignalType=real
  MATLAB Fcn1 : MATLABFcn  MATLABFcn=Ypoints(u(1))  OutputDimensions=1
  MATLAB Fcn2 : MATLABFcn  MATLABFcn=Zpoints(u(1))  OutputDimensions=1
  Mux : Mux  Inputs=3
  WP Coord : Outport
  wires:
  Data Type Conversion/1 -> MATLAB Fcn2/1, MATLAB Fcn/1, MATLAB Fcn1/1
  MATLAB Fcn/1 -> Mux/1
  MATLAB Fcn1/1 -> Mux/2
  MATLAB Fcn2/1 -> Mux/3
  WP Idx/1 -> Data Type Conversion/1
  Mux/1 -> Data Type Conversion1/1
  Data Type Conversion1/1 -> WP Coord/1

== system InnerOuter_Sim_newNav_flightgear_L2/L1 Output Feedback Controller With  Projection Operator/Control  Law ==
  a : Inport
  u : Inport  Port=2
  Compute Coef : Subsystem
  Detect Change : Subsystem
  Divide : Product  SampleTime=apSampleTime
  Divide1 : Product  SampleTime=apSampleTime
  IC : InitialCondition
  Integer Delay : Delay  DelayLength=1  InputProcessing=Inherited  SampleTime=apSampleTime
  Integer Delay1 : Delay  DelayLength=1  InputProcessing=Inherited  SampleTime=apSampleTime
  Subtract : Sum  SampleTime=apSampleTime
  y : Outport
  wires:
  Integer Delay1/1 -> Divide1/2
  u/1 -> Integer Delay/1
  IC/1 -> Compute Coef/Enable
  Subtract/1 -> Integer Delay1/1, y/1
  Divide1/1 -> Subtract/2
  Divide/1 -> Subtract/1
  Integer Delay/1 -> Divide/2
  Detect Change/1(change?) -> IC/1
  Compute Coef/2(c) -> Divide1/1
  Compute Coef/1(b) -> Divide/1
  a/1 -> Detect Change/1(Data), Compute Coef/1(a)

== system InnerOuter_Sim_newNav_flightgear_L2/L1 Output Feedback Controller With  Projection Operator/Projection Operator ==
  Theta Max : Inport
  Eps 0 : Inport  Port=2
  Theta : Inport  Port=3
  y : Inport  Port=4
  Compare To Zero : simulink/Logic and Bit Operations/Compare To Zero  relop=>=  OutDataTypeStr=boolean  ZeroCross=off
  Compare To Zero1 : simulink/Logic and Bit Operations/Compare To Zero  relop=>  OutDataTypeStr=boolean  ZeroCross=off
  Data Type Conversion1 : DataTypeConversion
  Divide2 : Product  OutDataTypeStr=single
  Enabled Subsystem : Subsystem  TreatAsAtomicUnit=on
  Enabled Subsystem1 : Subsystem  TreatAsAtomicUnit=on
  Enabled Subsystem2 : Subsystem  TreatAsAtomicUnit=on
  F(theta) : Subsystem
  Logical Operator : Logic  Operator=NOT  AllPortsSameDT=off  OutDataTypeStr=uint(8)
  Logical Operator2 : Logic  AllPortsSameDT=off  OutDataTypeStr=uint(8)
  Merge : Merge  InitialOutput=0
  Scope1 : Scope  NumInputPorts=4
      settings: YMin=-0.6~-0.5~-100~-10  YMax=0~5~10~10  SaveName=ScopeData4
  Scope2 : Scope  NumInputPorts=2
      settings: TimeRange=400  YMin=-0.06~-0.06  YMax=0.06~0.06  SaveName=ScopeData15
  "y " : InportShadow  Port=4
  "y    " : InportShadow  Port=4
  "Proj(the, y)" : Outport
  wires:
  Enabled Subsystem1/1(Out1) -> Merge/2
  "y    "/1 -> Enabled Subsystem1/1(y), Enabled Subsystem2/1(y), Scope1/2
  Logical Operator/1 -> Enabled Subsystem/Enable, Scope2/2
  Logical Operator2/1 -> Logical Operator/1, Enabled Subsystem1/Enable, Enabled Subsystem2/Enable, Scope2/1
  Compare To Zero1/1 -> Logical Operator2/1
  F(theta)/2(dif_f_theta) -> Divide2/1, Enabled Subsystem1/3(grad), Enabled Subsystem2/3(grad), Scope1/4
  Compare To Zero/1 -> Logical Operator2/2
  Enabled Subsystem/1(Out1) -> Data Type Conversion1/1
  "y "/1 -> Enabled Subsystem/1(In1)
  Merge/1 -> "Proj(the, y)"/1
  Divide2/1 -> Compare To Zero1/1
  y/1 -> Divide2/2
  F(theta)/1(f_theta) -> Compare To Zero/1, Enabled Subsystem1/2(f_the), Enabled Subsystem2/2(f_the), Scope1/3
  Theta/1 -> F(theta)/3(Theta)
  Eps 0/1 -> F(theta)/2(Eps 0)
  Theta Max/1 -> F(theta)/1(Theta Max)
  Data Type Conversion1/1 -> Merge/1
  Enabled Subsystem2/1(Out1) -> Scope1/1

== system InnerOuter_Sim_newNav_flightgear_L2/L1 Output Feedback Controller With  Projection Operator/State Predictor ==
  a : Inport
  u : Inport  Port=2
  Compute Coef : Subsystem
  Detect Change : Subsystem
  Divide : Product  SampleTime=apSampleTime
  Divide1 : Product  SampleTime=apSampleTime
  IC : InitialCondition
  Integer Delay : Delay  DelayLength=1  InputProcessing=Inherited  SampleTime=apSampleTime
  Integer Delay1 : Delay  DelayLength=1  InputProcessing=Inherited  SampleTime=apSampleTime
  Subtract : Sum  SampleTime=apSampleTime
  y : Outport
  wires:
  a/1 -> Compute Coef/1(a), Detect Change/1(Data)
  Compute Coef/1(b) -> Divide/1
  Compute Coef/2(c) -> Divide1/1
  Detect Change/1(change?) -> IC/1
  Integer Delay/1 -> Divide/2
  Divide/1 -> Subtract/1
  Divide1/1 -> Subtract/2
  Subtract/1 -> y/1, Integer Delay1/1
  IC/1 -> Compute Coef/Enable
  u/1 -> Integer Delay/1
  Integer Delay1/1 -> Divide1/2

== system InnerOuter_Sim_newNav_flightgear_L2/L1 Output Feedback Controller With  Projection Operator/Trapezoidal Integrator ==
  x : Inport
  Reset : Inport  Port=2
  Constant : Constant  Value=1/3  OutDataTypeStr=single
  Constant1 : Constant  Value=4/3  OutDataTypeStr=single
  Constant2 : Constant  Value=T/2  OutDataTypeStr=single
  Constant3 : Constant  Value=1/3  OutDataTypeStr=single
  Constant5 : Constant  Value=0  OutDataTypeStr=single
  Integer Delay : Delay  DelayLength=1  InputProcessing=Inherited  SampleTime=T
  Integer Delay1 : Delay  InputProcessing=Inherited  SampleTime=T
  Integer Delay2 : Delay  DelayLength=1  InputProcessing=Inherited  SampleTime=T
  Product{,1..3} (4 alike) : Product  OutDataTypeStr=single  RndMeth=Zero
  Protect NaNs : Subsystem
  Protect NaNs1 : Subsystem
  Subtract : Sum  Inputs=3  OutDataTypeStr=single
  Subtract1 : Sum  Inputs=2  OutDataTypeStr=single
  Switch1 : Switch  Criteria=u2 > Threshold  Threshold=0.3  SampleTime=.01
  "[min max]" : Saturate  UpperLimit=upperLimit  LowerLimit=lowerLimit  SampleTime=T
  Int(x) : Outport
  wires:
  Protect NaNs1/1(Out1) -> Integer Delay2/1, Int(x)/1
  Protect NaNs/1(Out1) -> Integer Delay1/1, Integer Delay/1, Product/1
  Subtract1/1 -> "[min max]"/1
  Product3/1 -> Subtract1/2
  "[min max]"/1 -> Switch1/3
  Switch1/1 -> Protect NaNs1/1(In1)
  Reset/1 -> Switch1/2
  Constant5/1 -> Switch1/1
  Integer Delay2/1 -> Subtract1/1
  Subtract/1 -> Product3/2
  Constant2/1 -> Product3/1
  Product2/1 -> Subtract/3
  Product1/1 -> Subtract/2
  Product/1 -> Subtract/1
  x/1 -> Protect NaNs/1(In1)
  Constant3/1 -> Product2/2
  Integer Delay1/1 -> Product2/1
  Integer Delay/1 -> Product1/1
  Constant1/1 -> Product1/2
  Constant/1 -> Product/2

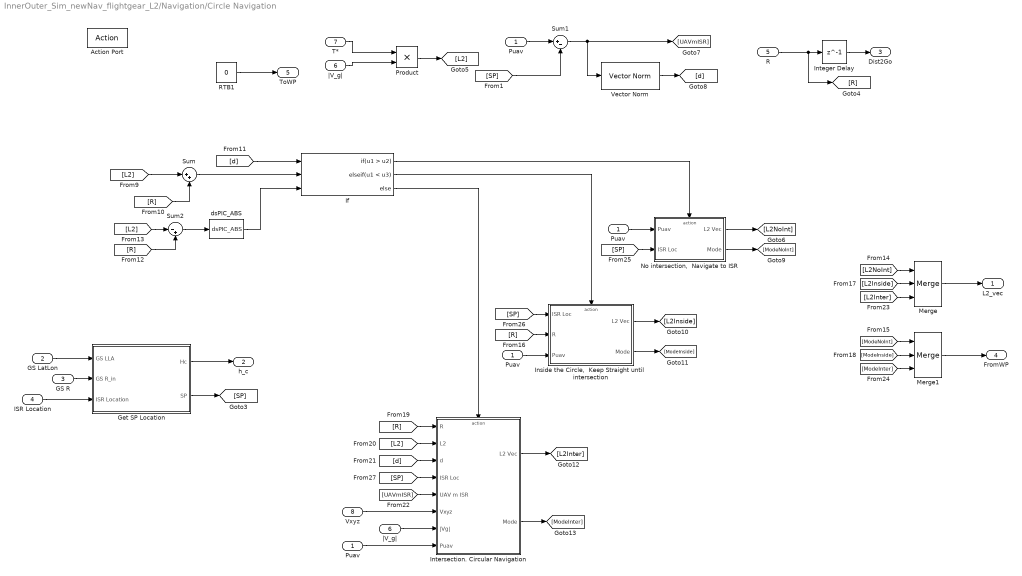
== system InnerOuter_Sim_newNav_flightgear_L2/Navigation/Circle Navigation ==
  Puav : Inport
  GS LatLon : Inport  Port=2
  GS R : Inport  Port=3
  ISR Location : Inport  Port=4
  R : Inport  Port=5
  |V_g| : Inport  Port=6
  T* : Inport  Port=7
  Vxyz : Inport  Port=8
  Action Port : ActionPort  ActionType=elseif
  Get SP Location : Subsystem
  If : If  NumInputs=3  IfExpression=u1 > u2  ElseIfExpressions=u1 < u3
  "Inside the Circle,  Keep Straight until  intersection" : Subsystem  TreatAsAtomicUnit=on
  Integer Delay : Delay  DelayLength=1  InputProcessing=Inherited
  Intersection. Circular Navigation : Subsystem  TreatAsAtomicUnit=on
  Merge : Merge  Inputs=3
  Merge1 : Merge  Inputs=3
  "No intersection,  Navigate to ISR" : Subsystem  TreatAsAtomicUnit=on
  Product : Product  OutDataTypeStr=single  RndMeth=Zero
  "Puav   " : InportShadow  Port=1
  "Puav    " : InportShadow  Port=1
  "Puav     " : InportShadow  Port=1
  RTB1 : Constant  Value=0  OutDataTypeStr=uint8
  Sum : Sum  Inputs=|++
  Sum1 : Sum  Inputs=|+-
  Sum2 : Sum  Inputs=|-+
  Vector Norm : SLUGS_Library/Vector Norm
  dsPIC_ABS : SLUGS_Library/dsPIC_ABS
  "|V_g| " : InportShadow  Port=6
  L2_vec : Outport
  h_c : Outport  Port=2
  Dist2Go : Outport  Port=3
  FromWP : Outport  Port=4  InitialOutput=[1]
  ToWP : Outport  Port=5  InitialOutput=[1]
  wires:
  Merge1/1 -> FromWP/1
  R/1 -> [R], Integer Delay/1
  Integer Delay/1 -> Dist2Go/1
  ISR Location/1 -> Get SP Location/3(ISR Location)
  GS R/1 -> Get SP Location/2(GS R_in)
  GS LatLon/1 -> Get SP Location/1(GS LLA)
  Get SP Location/2(SP) -> [SP]
  Product/1 -> [L2]
  |V_g|/1 -> Product/2
  T*/1 -> Product/1
  RTB1/1 -> ToWP/1
  [L2] -> Sum/1
  [R] -> Sum/2
  "Puav   "/1 -> Sum1/1
  [SP] -> Sum1/2
  Sum1/1 -> Vector Norm/1, [UAVmISR]
  Vector Norm/1 -> [d]
  [d] -> If/1
  Sum/1 -> If/2
  [L2] -> Sum2/1
  [R] -> Sum2/2
  Sum2/1 -> dsPIC_ABS/1
  dsPIC_ABS/1 -> If/3
  Merge/1 -> L2_vec/1
  If/1 -> "No intersection,  Navigate to ISR"/Action
  If/2 -> "Inside the Circle,  Keep Straight until  intersection"/Action
  If/3 -> Intersection. Circular Navigation/Action
  "Puav    "/1 -> "No intersection,  Navigate to ISR"/1(Puav)
  [SP] -> "No intersection,  Navigate to ISR"/2(ISR Loc)
  "No intersection,  Navigate to ISR"/1(L2 Vec) -> [L2NoInt]
  "No intersection,  Navigate to ISR"/2(Mode) -> [ModeNoInt]
  [L2NoInt] -> Merge/1
  [ModeNoInt] -> Merge1/1
  [SP] -> "Inside the Circle,  Keep Straight until  intersection"/1(ISR Loc)
  [R] -> "Inside the Circle,  Keep Straight until  intersection"/2(R)
  "Inside the Circle,  Keep Straight until  intersection"/1(L2 Vec) -> [L2Inside]
  "Inside the Circle,  Keep Straight until  intersection"/2(Mode) -> [ModeInside]
  [L2Inside] -> Merge/2
  [ModeInside] -> Merge1/2
  Puav/1 -> "Inside the Circle,  Keep Straight until  intersection"/3(Puav)
  Intersection. Circular Navigation/1(L2 Vec) -> [L2Inter]
  Intersection. Circular Navigation/2(Mode) -> [ModeInter]
  [R] -> Intersection. Circular Navigation/1(R)
  [L2] -> Intersection. Circular Navigation/2(L2)
  [d] -> Intersection. Circular Navigation/3(d)
  [SP] -> Intersection. Circular Navigation/4(ISR Loc)
  [UAVmISR] -> Intersection. Circular Navigation/5(UAV m ISR)
  Vxyz/1 -> Intersection. Circular Navigation/6(Vxyz)
  "|V_g| "/1 -> Intersection. Circular Navigation/7(|Vg|)
  [L2Inter] -> Merge/3
  [ModeInter] -> Merge1/3
  Get SP Location/1(Hc) -> h_c/1
  "Puav     "/1 -> Intersection. Circular Navigation/8(Puav)

== system InnerOuter_Sim_newNav_flightgear_L2/Navigation/Get 2D Groundspeed ==
  Vxyz : Inport  SampleTime=apSampleTime
  Vector Norm : SLUGS_Library/Vector Norm
  |V_g| : Outport
  wires:
  Vxyz/1 -> Vector Norm/1
  Vector Norm/1 -> |V_g|/1

== system InnerOuter_Sim_newNav_flightgear_L2/Navigation/L2+ ==
  |V_g| : Inport
  L2_vec : Inport  Port=2
  Vxyz : Inport  Port=3
  T*(m) : Inport  Port=4
  Constant10 : Constant  Value=maxEta  OutDataTypeStr=single
  "Get Sin, Cos eta" : Subsystem
  L2+ : Subsystem
  Rad2Deg : Gain  Gain=180/pi
  Relational Operator : RelationalOperator  Operator=<=  OutDataTypeStr=boolean
  Subsystem : Subsystem
  Switch : Switch  Criteria=u2 > Threshold  Threshold=0.3
  dsPIC_ABS : SLUGS_Library/dsPIC_ABS
  dsPIC_atan2 : SLUGS_Library/dsPIC_atan2
  "if sin(eta) < 0 - maxAcc else                 maxAcc " : Subsystem
  "|V_g| " : InportShadow  Port=1
  phi_c : Outport
  eta : Outport  Port=2
  wires:
  Vxyz/1 -> "Get Sin, Cos eta"/3(Vxyz)
  L2_vec/1 -> "Get Sin, Cos eta"/2(L2_vec)
  |V_g|/1 -> "Get Sin, Cos eta"/1(|V_g|)
  Switch/1 -> Subsystem/1(a_c)
  "if sin(eta) < 0 - maxAcc else                 maxAcc "/1(+ - maxAcc) -> Switch/3
  L2+/1(a_c) -> Switch/1
  Relational Operator/1 -> Switch/2
  Constant10/1 -> Relational Operator/2
  dsPIC_ABS/1 -> Relational Operator/1
  dsPIC_atan2/1 -> dsPIC_ABS/1, Rad2Deg/1  "eta"
  "Get Sin, Cos eta"/2(cos(eta)) -> dsPIC_atan2/2
  "Get Sin, Cos eta"/1(sin(eta)) -> "if sin(eta) < 0 - maxAcc else                 maxAcc "/1(sin(eta)), dsPIC_atan2/1, L2+/1(sin(eta))
  "|V_g| "/1 -> L2+/2(|V_g|)
  T*(m)/1 -> L2+/3(T*)
  Subsystem/1(phi_c) -> phi_c/1
  Rad2Deg/1 -> eta/1

== system InnerOuter_Sim_newNav_flightgear_L2/Navigation/Line Segment ==
  Puav : Inport
  MidLvl h_c : Inport  Port=2
  Action Port : ActionPort  ActionType=elseif
  Gain : Gain  Gain=-1
  Gain1 : Gain  Gain=-1
  "Puav " : InportShadow  Port=1
  RTB : Constant  Value=0  OutDataTypeStr=uint8
  RTB1 : Constant  Value=0  OutDataTypeStr=uint8
  Vector Norm : SLUGS_Library/Vector Norm
  L2_vec : Outport
  h_c : Outport  Port=2
  Dist2Go : Outport  Port=3
  FromWP : Outport  Port=4  InitialOutput=[1]
  ToWP : Outport  Port=5  InitialOutput=[2]
  wires:
  RTB1/1 -> ToWP/1
  Gain1/1 -> Vector Norm/1
  "Puav "/1 -> Gain1/1
  RTB/1 -> FromWP/1
  Vector Norm/1 -> Dist2Go/1
  MidLvl h_c/1 -> h_c/1
  Puav/1 -> Gain/1
  Gain/1 -> L2_vec/1

== system InnerOuter_Sim_newNav_flightgear_L2/Navigation/Minimum Turn Radius ==
  U_c : Inport
  Scale Factor : Inport  Port=2
  Constant1 : Constant  Value=maxAcc  OutDataTypeStr=single
  IC : InitialCondition  Value=1.5
  Product1 : Product  RndMeth=Zero
  Product2 : Product  RndMeth=Zero
  Product3 : Product  Inputs=*/  RndMeth=Zero
  "[1.5 10]" : Saturate  UpperLimit=10  LowerLimit=1.5
  R : Outport
  wires:
  IC/1 -> "[1.5 10]"/1
  "[1.5 10]"/1 -> Product2/1
  Product3/1 -> R/1
  Scale Factor/1 -> IC/1
  Product1/1 -> Product2/2
  Constant1/1 -> Product3/2
  Product2/1 -> Product3/1
  U_c/1 -> Product1/1, Product1/2
